simulink model "multi_input_regulator_firstpoles_firststructure"  (R2021b)
settings: Solver=VariableStepAuto  StartTime=0.0  StopTime=3  RelTol=1e-3
undefined symbols (not defined in the file): A, B_B, C, ks1_1
settings Model: Creator=nima8  LastModifiedBy=nima8

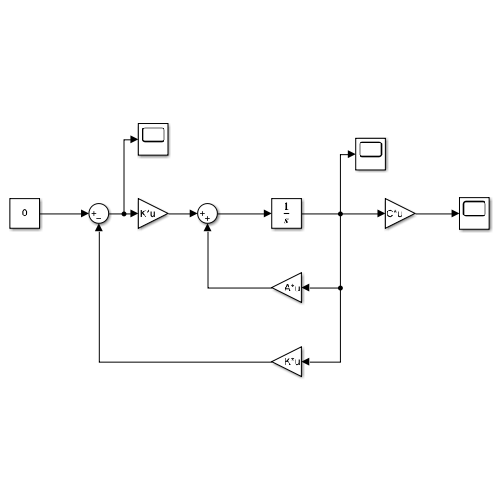
[thumbnail: Simulink's stored preview of the top-level diagram]
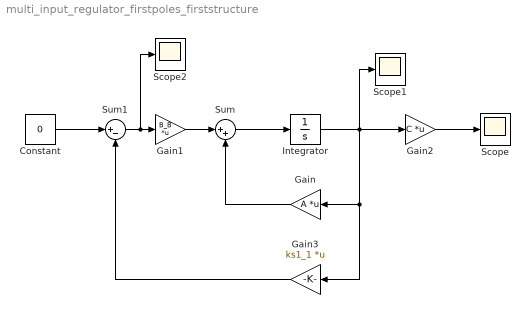
== system multi_input_regulator_firstpoles_firststructure ==
  Constant : Constant  Value=0
  Gain : Gain  Gain=A  Multiplication=Matrix(K*u)
  Gain1 : Gain  Gain=B_B  Multiplication=Matrix(K*u)
  Gain2 : Gain  Gain=C  Multiplication=Matrix(K*u)
  Gain3 : Gain  Gain=ks1_1  Multiplication=Matrix(K*u)
  Integrator : Integrator  InitialCondition=[1 0.5 -1 2]
  Scope : Scope
  Scope1 : Scope
  Scope2 : Scope
  Sum : Sum  Inputs=|++
  Sum1 : Sum  Inputs=|+-
  wires:
  Sum/1 -> Integrator/1
  Gain/1 -> Sum/2
  Gain2/1 -> Scope/1
  Integrator/1 -> Scope1/1, Gain/1, Gain3/1, Gain2/1
  Gain1/1 -> Sum/1
  Gain3/1 -> Sum1/2
  Sum1/1 -> Scope2/1, Gain1/1
  Constant/1 -> Sum1/1
